simulink model "TMPdemo"  (Simulink 6.0)
settings: Solver=ode45  StartTime=0.0  StopTime=100  RelTol=1e-3
PreLoadFcn:
  | mpctmpinit
values from neighbouring files (symbols this model uses):
  Fb0 = -(Cp0^2)/vp0/Gcd    (= 3.55555555556)    [mpctmpinit.m]
  Fbh0 = (ke*mlp0-dp0+vp0*Fb0/Cp0)/vp0    (= 6.82828282828)    [mpctmpinit.m]
  ke = -(dp0-((vp0/Cp0)^2)*Fb0*Gcv)/(mlp0-vp0*Glv)    (= 12.7272727273)    [mpctmpinit.m]
  ke2 = -((m2/Cs0)-M2-ds0)/mls0    (= 12.2245913291)    [mpctmpinit.m]
  kf = mlp0/(vp0*Fb0*Cp0*(1.2-0.3*gp0))    (= 0.20751953125)    [mpctmpinit.m]
  kf2 = mls0/(m2*Cs0*(1.2-0.3*gs0))    (= 0.170918367347)    [mpctmpinit.m]
  m2 = vp0*Fb0    (= 106.666666667)    [mpctmpinit.m]
  M2 = vp0*Fbh0+dp0-ke*mlp0    (= 266.666666667)    [mpctmpinit.m]
libraries: cstblocks x9, simulink x4, mpclib x1
settings Model: Creator=jowen  LastModifiedBy=jowen
settings DataIOCC: SaveFinalState=on  SignalLoggingName=logsOut
settings DebuggingCC: CheckExecutionContextPreStartOutputMsg=on  CheckExecutionContextRuntimeOutputMsg=on
settings SFSimCC: SFSimApplyToAllLibs=on  SFSimBuildMode=Incremental

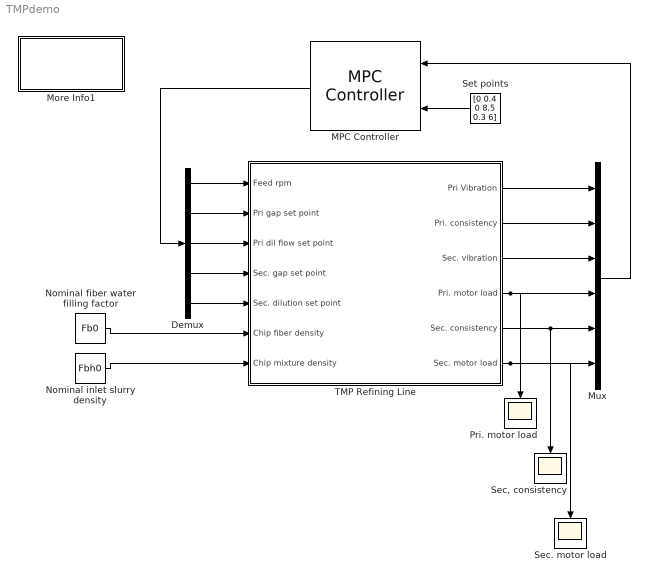
== system TMPdemo ==
  Demux : Demux  Outputs=5
  MPC Controller : mpclib/MPC Controller  Orientation=left  mpcobj=MPC1  n_mv=0  x0=[]  ref_from_ws=off  ref_signal_name=[]  ref_preview=on  md_from_ws=off  md_signal_name=[]  md_preview=on  from_project=off  md_inport=off  project_file=MPCtask.mat
  More Info1 : Subsystem  PropExecContextAcrossSSBoundary=on
      settings: OpenFcn=mpcdesign_callback(gcs);
      mask Display: disp('Double click\nhere to\nStart')
  Mux : Mux  Inputs=6
  Nominal fiber water filling factor : Constant  Value=Fb0
  Nominal inlet slurry density : Constant  Value=Fbh0
  Pri. motor load : Scope
      settings: Orientation=down  YMin=0.3825  YMax=0.415
  "Sec, consistency" : Scope
      settings: Orientation=down  YMin=0.3825  YMax=0.415
  Sec. motor load : Scope
      settings: Orientation=down  YMin=0.3825  YMax=0.415  SaveName=ScopeData2
  Set points : Constant  Orientation=left  Value=[0 0.4 0 8.5 0.3 6]
  TMP Refining Line : Subsystem  PropExecContextAcrossSSBoundary=on
  wires:
  Demux/1 -> TMP Refining Line/1(Feed rpm)
  Demux/3 -> TMP Refining Line/3(Pri dil flow set point)
  Demux/4 -> TMP Refining Line/4(Sec. gap set point)
  Demux/5 -> TMP Refining Line/5(Sec. dilution set point)
  TMP Refining Line/1(Pri Vibration) -> Mux/1
  TMP Refining Line/2(Pri. consistency) -> Mux/2
  TMP Refining Line/3(Sec. vibration) -> Mux/3
  TMP Refining Line/4(Pri. motor load) -> Mux/4, Pri. motor load/1
  TMP Refining Line/5(Sec. consistency) -> Mux/5, "Sec, consistency"/1
  TMP Refining Line/6(Sec. motor load) -> Mux/6, Sec. motor load/1
  Mux/1 -> MPC Controller/1
  Set points/1 -> MPC Controller/2
  Demux/2 -> TMP Refining Line/2(Pri gap set point)
  Nominal fiber water filling factor/1 -> TMP Refining Line/6(Chip fiber density)
  MPC Controller/1 -> Demux/1
  Nominal inlet slurry density/1 -> TMP Refining Line/7(Chip mixture density)

== system TMPdemo/More Info1 ==

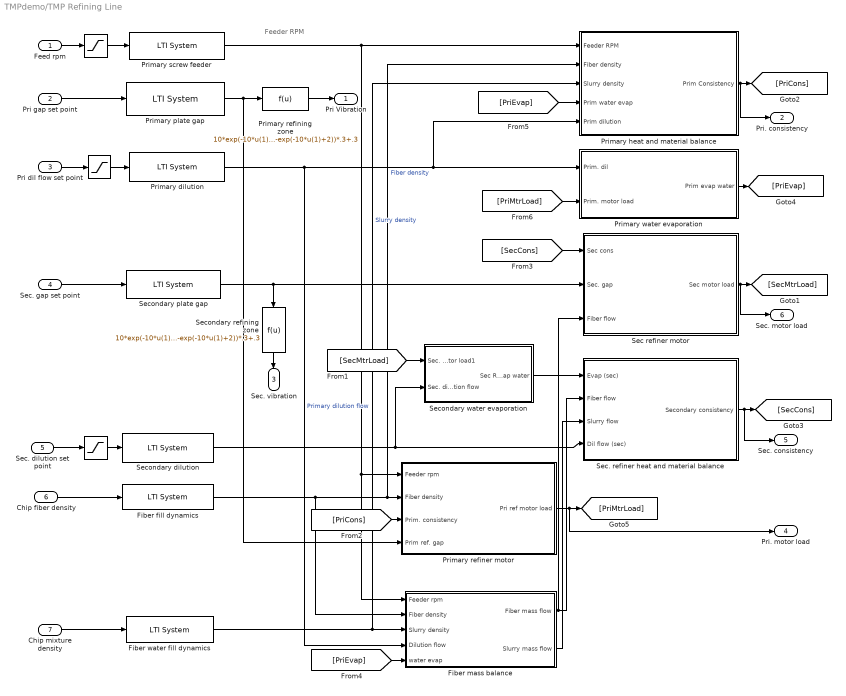
== system TMPdemo/TMP Refining Line ==
  note: Feeder RPM
  Feed rpm : Inport  LatchInput=off
  Pri gap set point : Inport  Port=2  LatchInput=off
  Pri dil flow set point : Inport  Port=3  LatchInput=off
  Sec. gap set point : Inport  Port=4  LatchInput=off
  Sec. dilution set point : Inport  Port=5  LatchInput=off
  Chip fiber density : Inport  Port=6  LatchInput=off
  Chip mixture density : Inport  Port=7  LatchInput=off
  "  " : Saturate  UpperLimit=35  LowerLimit=25  SampleTime=0.5
  "    " : Saturate  UpperLimit=200  LowerLimit=90  SampleTime=0.5
  "       " : Saturate  UpperLimit=200  LowerLimit=90  SampleTime=0.5
  Fiber fill dynamics : cstblocks/LTI System  sys=FiberFill  IC=Fb0
  Fiber mass balance : Subsystem  PropExecContextAcrossSSBoundary=on
  Fiber water fill dynamics : cstblocks/LTI System  sys=FiberWaterFill  IC=Fbh0
  Primary dilution : cstblocks/LTI System  sys=DilFlowPrimary  IC=dp0
  Primary heat and material balance : Subsystem  PropExecContextAcrossSSBoundary=on
  Primary plate gap : cstblocks/LTI System  sys=PlateGapPrimary  IC=gp0
  Primary refiner motor : Subsystem  PropExecContextAcrossSSBoundary=on
  Primary refining zone : Fcn  Expr=10*exp(-10*u(1)+2)*(1.26-0.3*u(1))-(1-exp(-10*u(1)+2))*.3+.3
  Primary screw feeder : cstblocks/LTI System  sys=ChipFeeder  IC=vp0
  Primary water evaporation : Subsystem  PropExecContextAcrossSSBoundary=on
  Sec refiner motor : Subsystem  PropExecContextAcrossSSBoundary=on
  Sec. refiner heat and material balance : Subsystem  PropExecContextAcrossSSBoundary=on
  "Secondary dilution " : cstblocks/LTI System  sys=DilFlowSecondary  IC=gs0
  Secondary plate gap : cstblocks/LTI System  sys=PlateGapSecondary  IC=gs0
  Secondary refining zone : Fcn  Orientation=down  Expr=10*exp(-10*u(1)+2)*(1.26-0.3*u(1))-(1-exp(-10*u(1)+2))*.3+.3  SampleTime=0.5
  Secondary water evaporation : Subsystem  PropExecContextAcrossSSBoundary=on
  Pri Vibration : Outport
  Pri. consistency : Outport  Port=2
  Sec. vibration : Outport  Orientation=down  Port=3
  Pri. motor load : Outport  Port=4
  Sec. consistency : Outport  Port=5
  Sec. motor load : Outport  Port=6
  wires:
  "  "/1 -> Primary screw feeder/1
  Primary plate gap/1 -> Primary refining zone/1, Primary refiner motor/4(Prim ref. gap)
  Secondary plate gap/1 -> Secondary refining zone/1, Sec refiner motor/2(Sec. gap)
  "    "/1 -> Primary dilution/1
  "       "/1 -> "Secondary dilution "/1
  "Secondary dilution "/1 -> Sec. refiner heat and material balance/4(Dil flow (sec)), Secondary water evaporation/2(Sec. dilution flow)
  Sec. dilution set point/1 -> "       "/1
  Fiber water fill dynamics/1 -> Primary heat and material balance/3(Slurry density), Fiber mass balance/3(Slurry density)  "Slurry density"
  Fiber fill dynamics/1 -> Fiber mass balance/2(Fiber density), Primary heat and material balance/2(Fiber density), Primary refiner motor/2(Fiber density)  "Fiber density"
  Primary dilution/1 -> Primary water evaporation/1(Prim. dil), Primary heat and material balance/5(Prim dilution), Fiber mass balance/4(Dilution flow)  "Primary dilution flow"
  Primary screw feeder/1 -> Primary heat and material balance/1(Feeder RPM), Fiber mass balance/1(Feeder rpm), Primary refiner motor/1(Feeder rpm)
  Fiber mass balance/1(Fiber mass flow) -> Sec. refiner heat and material balance/2(Fiber flow), Sec refiner motor/3(Fiber flow)
  Fiber mass balance/2(Slurry mass flow) -> Sec. refiner heat and material balance/3(Slurry flow)
  Secondary water evaporation/1(Sec Ref. evap water) -> Sec. refiner heat and material balance/1(Evap (sec))
  Primary refining zone/1 -> Pri Vibration/1
  Sec refiner motor/1(Sec motor load) -> [SecMtrLoad], Sec. motor load/1
  Primary heat and material balance/1(Prim Consistency) -> [PriCons], Pri. consistency/1
  [PriCons] -> Primary refiner motor/3(Prim. consistency)
  Sec. refiner heat and material balance/1(Secondary consistency) -> [SecCons], Sec. consistency/1
  [SecCons] -> Sec refiner motor/1(Sec cons)
  Primary water evaporation/1(Prim evap water) -> [PriEvap]
  [PriEvap] -> Primary heat and material balance/4(Prim water evap)
  Primary refiner motor/1(Pri ref motor load) -> [PriMtrLoad], Pri. motor load/1
  [PriMtrLoad] -> Primary water evaporation/2(Prim. motor load)
  [SecMtrLoad] -> Secondary water evaporation/1(Sec. motor load1)
  Feed rpm/1 -> "  "/1
  Pri gap set point/1 -> Primary plate gap/1
  Pri dil flow set point/1 -> "    "/1
  Sec. gap set point/1 -> Secondary plate gap/1
  Secondary refining zone/1 -> Sec. vibration/1
  [PriEvap] -> Fiber mass balance/5(water evap)
  Chip fiber density/1 -> Fiber fill dynamics/1
  Chip mixture density/1 -> Fiber water fill dynamics/1

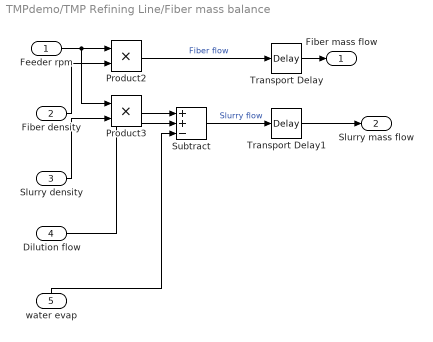
== system TMPdemo/TMP Refining Line/Fiber mass balance ==
  Feeder rpm : Inport  LatchInput=off
  Fiber density : Inport  Port=2  LatchInput=off
  Slurry density : Inport  Port=3  LatchInput=off
  Dilution flow : Inport  Port=4  LatchInput=off
  water evap : Inport  Orientation=up  Port=5  LatchInput=off
  Product2 : Product  RndMeth=Zero
  Product3 : Product  RndMeth=Zero
  Subtract : Sum  Inputs=++-  OutScaling=2^-10
  Transport Delay : TransportDelay  DelayTime=2  InitialInput=m2
  Transport Delay1 : TransportDelay  DelayTime=2  InitialInput=M2
  Fiber mass flow : Outport
  Slurry mass flow : Outport  Port=2
  wires:
  Product2/1 -> Transport Delay/1  "Fiber flow"
  Product3/1 -> Subtract/1
  Subtract/1 -> Transport Delay1/1  "Slurry flow"
  Feeder rpm/1 -> Product2/1, Product3/1
  Fiber density/1 -> Product2/2
  Slurry density/1 -> Product3/2
  Dilution flow/1 -> Subtract/2
  water evap/1 -> Subtract/3
  Transport Delay/1 -> Fiber mass flow/1
  Transport Delay1/1 -> Slurry mass flow/1

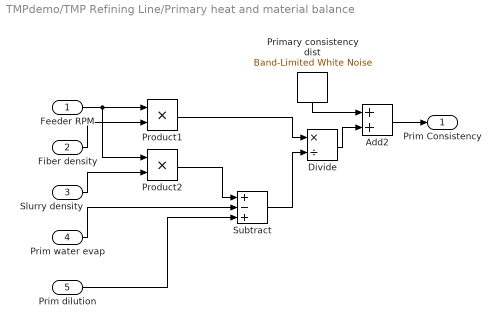
== system TMPdemo/TMP Refining Line/Primary heat and material balance ==
  Feeder RPM : Inport  LatchInput=off
  Fiber density : Inport  Port=2  LatchInput=off
  Slurry density : Inport  Port=3  LatchInput=off
  Prim water evap : Inport  Port=4  LatchInput=off
  Prim dilution : Inport  Port=5  LatchInput=off
  Add2 : Sum  OutScaling=2^-10
  Divide : Product  Inputs=*/  OutScaling=2^-10  SampleTime=.5
  Primary consistency dist : simulink/Sources/Band-Limited White Noise  Orientation=down  Cov=0.00001  Ts=0.5  seed=[23341]
  Product1 : Product  RndMeth=Zero
  Product2 : Product  RndMeth=Zero
  Subtract : Sum  Inputs=+-+  OutScaling=2^-10
  Prim Consistency : Outport
  wires:
  Product2/1 -> Subtract/1
  Subtract/1 -> Divide/2
  Product1/1 -> Divide/1
  Divide/1 -> Add2/2
  Primary consistency dist/1 -> Add2/1
  Feeder RPM/1 -> Product1/1, Product2/1
  Prim dilution/1 -> Subtract/3
  Add2/1 -> Prim Consistency/1
  Fiber density/1 -> Product1/2
  Slurry density/1 -> Product2/2
  Prim water evap/1 -> Subtract/2

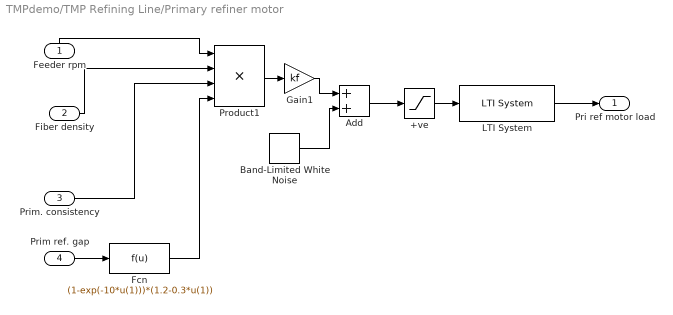
== system TMPdemo/TMP Refining Line/Primary refiner motor ==
  Feeder rpm : Inport  Orientation=up  LatchInput=off
  Fiber density : Inport  Port=2  LatchInput=off
  Prim. consistency : Inport  Port=3  LatchInput=off
  Prim ref. gap : Inport  Port=4  LatchInput=off
  +ve : Saturate  UpperLimit=inf  LowerLimit=0  SampleTime=0.5
  Add : Sum  OutScaling=2^-10
  Band-Limited White Noise : simulink/Sources/Band-Limited White Noise  Cov=0.0001  Ts=0.5  seed=[23341]
  Fcn : Fcn  Expr=(1-exp(-10*u(1)))*(1.2-0.3*u(1))
  Gain1 : Gain  Gain=kf
  LTI System : cstblocks/LTI System  sys=UnitDelay  IC=mlp0
  Product1 : Product  Inputs=4  RndMeth=Zero
  Pri ref motor load : Outport
  wires:
  Product1/1 -> Gain1/1
  Fcn/1 -> Product1/4
  Gain1/1 -> Add/1
  Add/1 -> +ve/1
  Band-Limited White Noise/1 -> Add/2
  Feeder rpm/1 -> Product1/1
  Fiber density/1 -> Product1/2
  Prim ref. gap/1 -> Fcn/1
  Prim. consistency/1 -> Product1/3
  +ve/1 -> LTI System/1
  LTI System/1 -> Pri ref motor load/1

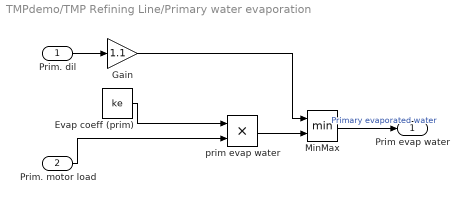
== system TMPdemo/TMP Refining Line/Primary water evaporation ==
  Prim. dil : Inport  LatchInput=off
  Prim. motor load : Inport  Port=2  LatchInput=off
  Evap coeff (prim) : Constant  Value=ke
  Gain : Gain  Gain=1.1
  MinMax : MinMax  Inputs=2
  prim evap water : Product  RndMeth=Zero
  Prim evap water : Outport
  wires:
  Evap coeff (prim)/1 -> prim evap water/1
  prim evap water/1 -> MinMax/2
  Gain/1 -> MinMax/1
  Prim. dil/1 -> Gain/1
  MinMax/1 -> Prim evap water/1  "Primary evaporated water"
  Prim. motor load/1 -> prim evap water/2

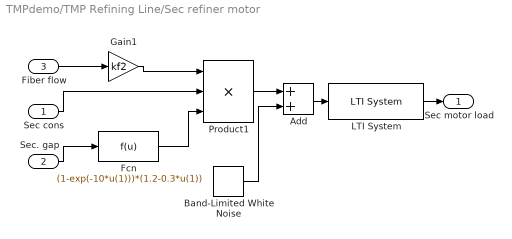
== system TMPdemo/TMP Refining Line/Sec refiner motor ==
  Sec cons : Inport  LatchInput=off
  Sec. gap : Inport  Port=2  LatchInput=off
  Fiber flow : Inport  Port=3  LatchInput=off
  Add : Sum  OutScaling=2^-10
  Band-Limited White Noise : simulink/Sources/Band-Limited White Noise  Cov=0.0001  Ts=0.5  seed=[23341]
  Fcn : Fcn  Expr=(1-exp(-10*u(1)))*(1.2-0.3*u(1))
  Gain1 : Gain  Gain=kf2
  LTI System : cstblocks/LTI System  sys=UnitDelay  IC=mls0
  Product1 : Product  Inputs=3  RndMeth=Zero
  Sec motor load : Outport
  wires:
  Gain1/1 -> Product1/1
  Fcn/1 -> Product1/3
  Product1/1 -> Add/1
  Band-Limited White Noise/1 -> Add/2
  Fiber flow/1 -> Gain1/1
  Sec. gap/1 -> Fcn/1
  Sec cons/1 -> Product1/2
  Add/1 -> LTI System/1
  LTI System/1 -> Sec motor load/1

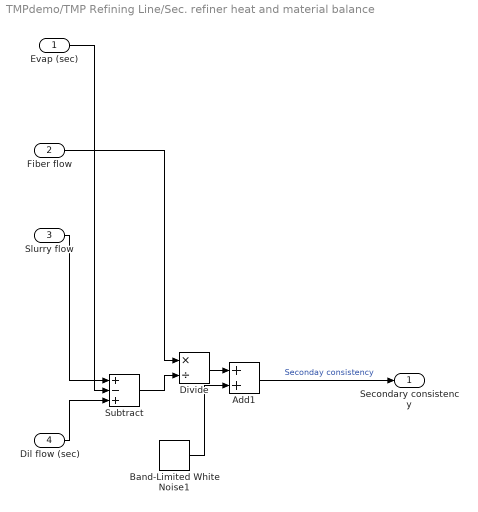
== system TMPdemo/TMP Refining Line/Sec. refiner heat and material balance ==
  Evap (sec) : Inport  LatchInput=off
  Fiber flow : Inport  Port=2  LatchInput=off
  Slurry flow : Inport  Port=3  LatchInput=off
  Dil flow (sec) : Inport  Port=4  LatchInput=off
  Add1 : Sum  OutScaling=2^-10
  Band-Limited White Noise1 : simulink/Sources/Band-Limited White Noise  Cov=0.00001  Ts=0.5  seed=[23341]
  Divide : Product  Inputs=*/  OutScaling=2^-10  SampleTime=.5
  Subtract : Sum  Inputs=+-+  OutScaling=2^-10
  Secondary consistency : Outport
  wires:
  Evap (sec)/1 -> Subtract/2
  Subtract/1 -> Divide/2
  Divide/1 -> Add1/1
  Band-Limited White Noise1/1 -> Add1/2
  Fiber flow/1 -> Divide/1
  Dil flow (sec)/1 -> Subtract/3
  Add1/1 -> Secondary consistency/1  "Seconday consistency"
  Slurry flow/1 -> Subtract/1

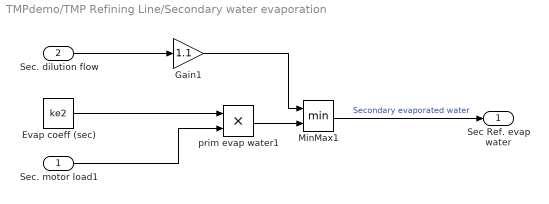
== system TMPdemo/TMP Refining Line/Secondary water evaporation ==
  Sec. motor load1 : Inport  LatchInput=off
  Sec. dilution flow : Inport  Port=2  LatchInput=off
  Evap coeff (sec) : Constant  Value=ke2
  Gain1 : Gain  Gain=1.1
  MinMax1 : MinMax  Inputs=2
  prim evap water1 : Product  RndMeth=Zero
  Sec Ref. evap water : Outport
  wires:
  Evap coeff (sec)/1 -> prim evap water1/1
  prim evap water1/1 -> MinMax1/2
  Sec. dilution flow/1 -> Gain1/1
  Sec. motor load1/1 -> prim evap water1/2
  Gain1/1 -> MinMax1/1
  MinMax1/1 -> Sec Ref. evap water/1  "Secondary evaporated water"
